simulink model "Actuateur"  (R2019b)
settings: Solver=VariableStepAuto  StartTime=0.0  StopTime=6  MaxStep=0.0001  RelTol=1e-3
settings Model: Creator=jeanz  LastModifiedBy=jeanz

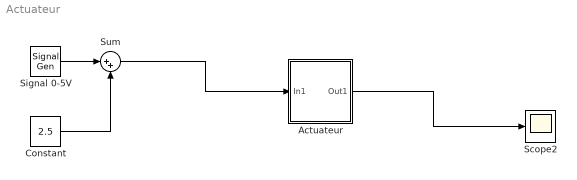
== system Actuateur ==
  Actuateur : Subsystem
  Constant : Constant  Value=2.5
  Scope2 : Scope
  Signal 0-5V : SignalGenerator  WaveForm=square  Amplitude=2.5  Frequency=10  Units=rad/sec
  Sum : Sum  Inputs=|++
  wires:
  Signal 0-5V/1 -> Sum/1
  Constant/1 -> Sum/2
  Sum/1 -> Actuateur/1(In1)
  Actuateur/1(Out1) -> Scope2/1

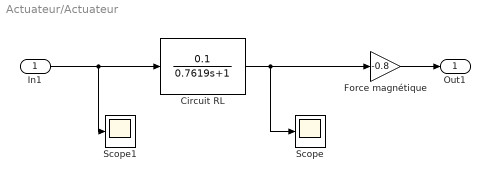
== system Actuateur/Actuateur ==
  In1 : Inport
  Circuit RL : TransferFcn  Numerator=[0.1]  Denominator=[0.7619 1]
  Force magnétique : Gain  Gain=-0.8
  Scope : Scope
  Scope1 : Scope
  Out1 : Outport
  wires:
  Force magnétique/1 -> Out1/1
  Circuit RL/1 -> Force magnétique/1, Scope/1
  In1/1 -> Scope1/1, Circuit RL/1
